simulink model "sampleModel6041_pp_1873_1_difftest"  (R2021a)
settings: Solver=VariableStepAuto  StartTime=0.0  StopTime=10.0  RelTol=1e-3
undefined symbols (not defined in the file or in its folder): Newton, Raphson
libraries: simulink x15, pid_lib x3
settings Model: Creator=O1  LastModifiedBy=user

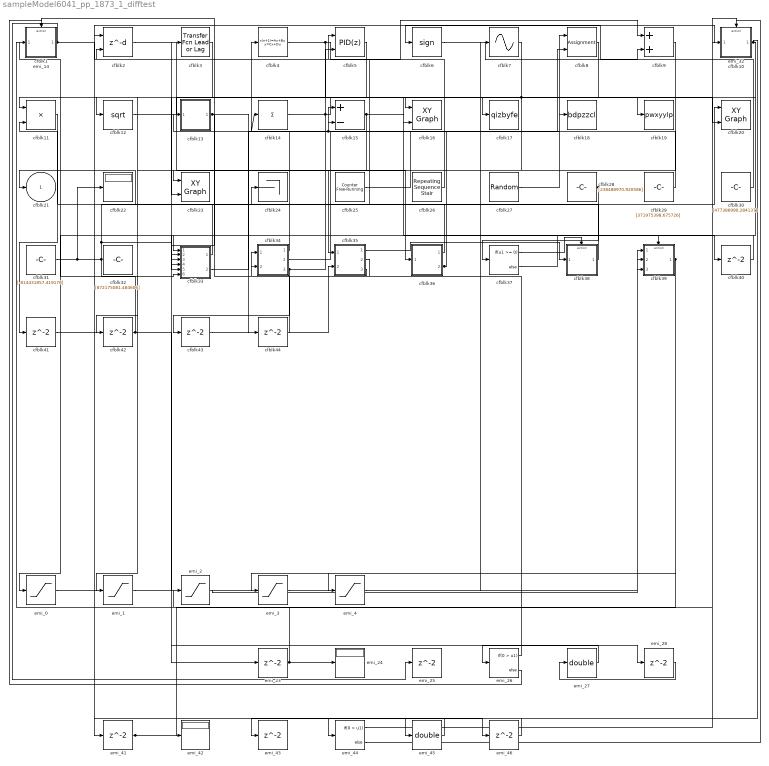
== system sampleModel6041_pp_1873_1_difftest ==
  cfblk1 : Subsystem  TreatAsAtomicUnit=on
  cfblk10 : Subsystem  TreatAsAtomicUnit=on
  cfblk11 : Product
  cfblk12 : Sqrt  SaturateOnIntegerOverflow=on
  cfblk13 : Subsystem  TreatAsAtomicUnit=on
  cfblk14 : Sum  Inputs=+
  cfblk15 : Sum  Inputs=+-
  cfblk16 : simulink/Sinks/XY Graph  xmin=-1  xmax=1  ymin=-1  ymax=1  st=-1
  cfblk17 : ToWorkspace  VariableName=qizbyfe  SaveFormat=Timeseries  SampleTime=-1
  cfblk18 : ToWorkspace  VariableName=bdpzzcl  SaveFormat=Timeseries  SampleTime=-1
  cfblk19 : ToWorkspace  VariableName=pwxyylp  SaveFormat=Timeseries  SampleTime=-1
  cfblk2 : Delay  DelayLengthSource=Input port  SampleTime=1
      settings: InputPortMap=u0,p1
  cfblk20 : simulink/Sinks/XY Graph  xmin=-1  xmax=1  ymin=-1  ymax=1  st=-1
  cfblk22 : Display
  cfblk23 : simulink/Sinks/XY Graph  xmin=-1  xmax=1  ymin=-1  ymax=1  st=-1
  cfblk24 : Terminator
  cfblk25 : simulink/Sources/Counter Free-Running  NumBits=[51.000000]  tsamp=-1
  cfblk26 : simulink/Sources/Repeating Sequence Stair  OutValues=[88415445.174803, 597697851.659731]  tsamp=-1  OutMin=[]  OutMax=[]  OutDataTypeStr=double  OutputDataTypeScalingMode=double  OutDataType=fixdt(0,8)  ConRadixGroup=Best Precision: Vector-wise  OutScaling=2^-12
  cfblk27 : RandomNumber  Mean=[16875.692149]  Variance=[94231.226590]  Seed=[933993458.000000]  SampleTime=0.1
  cfblk28 : Constant  Value=[238488970.920586]  SampleTime=1
  cfblk29 : Constant  Value=[371975398.675726]  SampleTime=1
  cfblk3 : simulink/Discrete/Transfer Fcn Lead or Lag  PoleZ=0.95  ZeroZ=0.75  ICPrevOutput=0.0  ICPrevInput=0.0  DoSatur=off
      settings: SourceProductBaseCode=SL
  cfblk30 : Constant  Value=[477386990.284137]  SampleTime=1
  cfblk31 : Constant  Value=[-814431857.419178]  SampleTime=1
  cfblk32 : Constant  Value=[872175081.484606]  SampleTime=1
  cfblk33 : Subsystem
  cfblk34 : Subsystem
  cfblk35 : Subsystem
  cfblk36 : Subsystem
  cfblk37 : If  IfExpression=u1 >= 0  SampleTime=1
  cfblk38 : Subsystem  TreatAsAtomicUnit=on
  cfblk39 : Subsystem  TreatAsAtomicUnit=on
  cfblk4 : DiscreteStateSpace
  cfblk{40..44} (5 alike) : Delay  SampleTime=1
  cfblk5 : pid_lib/PID Controller (2DOF)  Controller=PID  Form=Parallel  TimeDomain=Discrete-time  UseExternalTs=off  SampleTime=1  IntegratorMethod=Forward Euler  FilterMethod=Forward Euler  ControllerParametersSource=internal  P=1  I=1  D=0  UseFilter=on  N=100  b=1  c=1  TunerSelectOption=Transfer Function Based (PID Tuner App)  InitialConditionSource=internal  InitialConditionForIntegrator=0  InitialConditionForFilter=0  DifferentiatorICPrevScaledInput=0  ExternalReset=none  TrackingMode=off  Kt=1  LimitOutput=off  SatLimitsSource=internal  UpperSaturationLimit=inf  LowerSaturationLimit=-inf  LinearizeAsGain=off  AntiWindupMode=none  Kb=1  POutMin=[]  POutMax=[]  IOutMin=[]  IOutMax=[]  DOutMin=[]  DOutMax=[]  NOutMin=[]  NOutMax=[]  bOutMin=[]  bOutMax=[]  cOutMin=[]  cOutMax=[]  SumOutMin=[]  SumOutMax=[]  SaturationOutMin=[]  SaturationOutMax=[]  PParamMin=[]  PParamMax=[]  IParamMin=[]  IParamMax=[]  DParamMin=[]  DParamMax=[]  NParamMin=[]  NParamMax=[]  bParamMin=[]  bParamMax=[]  cParamMin=[]  cParamMax=[]  KbParamMin=[]  KbParamMax=[]  KtParamMin=[]  KtParamMax=[]  KbOutMin=[]  KbOutMax=[]  KtOutMin=[]  KtOutMax=[]  IntegratorOutMin=[]  IntegratorOutMax=[]  FilterOutMin=[]  FilterOutMax=[]  SumI1OutMin=[]  SumI1OutMax=[]  SumI2OutMin=[]  SumI2OutMax=[]  SumI3OutMin=[]  SumI3OutMax=[]  SumI4OutMin=[]  SumI4OutMax=[]  SumDOutMin=[]  SumDOutMax=[]  Sum1OutMin=[]  Sum1OutMax=[]  Sum2OutMin=[]  Sum2OutMax=[]  Sum3OutMin=[]  Sum3OutMax=[]  DifferentiatorOutMin=[]  DifferentiatorOutMax=[]  FilterDiffOutCoefMin=[]  FilterDiffOutCoefMax=[]  ReciprocalOutMin=[]  ReciprocalOutMax=[]  SumDenOutMin=[]  SumDenOutMax=[]  SumNumOutMin=[]  SumNumOutMax=[]  DivideOutMin=[]  DivideOutMax=[]  UdiffTsProdOutMin=[]  UdiffTsProdOutMax=[]  NTsProdOutMin=[]  NTsProdOutMax=[]  UintegralTsProdOutMin=[]  UintegralTsProdOutMax=[]  UngainTsProdOutMin=[]  UngainTsProdOutMax=[]  IntegratorContinuousStateAttributes=''  IntegratorStateMustResolveToSignalObject=off  IntegratorRTWStateStorageClass=Auto  FilterContinuousStateAttributes=''  FilterStateMustResolveToSignalObject=off  FilterRTWStateStorageClass=Auto  ParallelPVariant=InternalParameters  IdealPVariant=Disabled  IVariant=InternalParameters  DVariant=InternalParameters  bVariant=InternalParameters  cVariant=InternalParameters  IntegratorVariant=Discrete  SatVariant=Disabled  AWVariant=Passthrough  PCopyVariant=Disabled  TRVariant=Disabled  FdbkBlocksVariant=Forward  IdealPFdbkVariant=Disabled  SatFdbkVariant=Disabled  DerivativeFilterVariant=ForwardEulerFilter  NVariant=InternalParameters  NCopyVariant=Disabled  FilterICVariant=InternalICsFilter  IntegratorICVariant=InternalICs  ExternalResetVariant=Disabled  TRSumVariant=Passthrough  SumFdbkVariant=Disabled  SumVariant=Sum_PID  TsampFilterVariant=InternalTs  TsampNgainVariant=Passthrough  TsampIntegralVariant=Passthrough  ExternalSaturationOutDataTypeStr=Inherit: Same as second input
      settings: SourceProductBaseCode=SL
  cfblk6 : Signum
  cfblk7 : Sin  TimeSource=Use external signal  SampleTime=0
  cfblk8 : Assignment  DiagnosticForDimensions=Warning  IndexOptions=Index vector (dialog)  Indices=1  OutputSizes=1
  cfblk9 : Sum
  emi_{0..4} (5 alike) : Saturate  UpperLimit=0  LowerLimit=0  ZeroCross=off
  emi_14 : Subsystem  TreatAsAtomicUnit=on
  emi_{23,25,41,43} (4 alike) : Delay
  emi_24 : Display
  emi_26 : If  IfExpression=0 > u1
  emi_27 : DataTypeConversion  OutDataTypeStr=double
  emi_28 : Delay  InitialCondition=0
  emi_32 : Subsystem  TreatAsAtomicUnit=on
  emi_42 : Display
  emi_44 : If  IfExpression=0 > u1
  emi_45 : DataTypeConversion  OutDataTypeStr=double
  emi_46 : Delay  InitialCondition=0
  cfblk21 : Outport
  wires:
  cfblk8/1 -> cfblk11/1
  cfblk27/1 -> cfblk8/1
  cfblk7/1 -> cfblk23/1, cfblk16/2
  cfblk25/1 -> cfblk18/1
  cfblk34/1(cfblk2) -> cfblk4/1
  cfblk14/1 -> cfblk19/1, cfblk16/1
  cfblk35/1(cfblk2) -> cfblk38/1(cfblk1)
  cfblk2/1 -> cfblk36/1(cfblk1)
  cfblk30/1 -> cfblk6/1
  cfblk28/1 -> cfblk37/1, emi_0/1
  cfblk35/2(cfblk11) -> cfblk34/1(cfblk1)
  cfblk35/3(cfblk12) -> cfblk34/2(cfblk11)
  cfblk3/1 -> cfblk23/2
  cfblk4/1 -> cfblk9/1, cfblk20/2
  cfblk31/1 -> cfblk20/1, cfblk33/3(cfblk11), cfblk33/6(cfblk14), cfblk22/1
  cfblk33/1(cfblk2) -> cfblk21/1
  cfblk6/1 -> cfblk9/2
  cfblk33/2(cfblk15) -> cfblk15/1
  cfblk29/1 -> cfblk14/1, cfblk15/2
  cfblk36/1(cfblk2) -> cfblk5/1
  cfblk15/1 -> cfblk35/1(cfblk1), cfblk40/1
  cfblk38/1(cfblk2) -> cfblk11/2
  cfblk12/1 -> cfblk17/1
  cfblk34/2(cfblk12) -> cfblk8/2
  cfblk26/1 -> cfblk2/2
  cfblk34/3(cfblk13) -> cfblk5/2, cfblk43/1
  cfblk36/2(cfblk12) -> cfblk24/1, cfblk13/1(emi_9)
  cfblk37/1 -> cfblk38/Action
  cfblk37/2 -> cfblk39/Action
  cfblk40/1 -> cfblk33/1(cfblk1)
  cfblk11/1 -> cfblk41/1
  cfblk41/1 -> cfblk33/2(cfblk10)
  cfblk5/1 -> cfblk42/1
  cfblk43/1 -> cfblk35/2(cfblk10)
  cfblk44/1 -> cfblk2/1
  emi_0/1 -> cfblk7/1
  emi_1/1 -> cfblk3/1
  cfblk9/1 -> emi_1/1
  emi_2/1 -> cfblk39/1(cfblk1)
  cfblk39/1(cfblk2) -> emi_2/1, emi_3/1, emi_4/1
  emi_3/1 -> cfblk39/2(cfblk7)
  emi_4/1 -> cfblk39/3(cfblk8)
  cfblk13/1(emi_10) -> cfblk44/1, cfblk33/4(cfblk12)
  cfblk42/1 -> cfblk1/1(emi_12), emi_23/1, emi_28/1
  emi_23/1 -> emi_14/1(emi_21), emi_24/1
  emi_14/1(emi_22) -> emi_25/1
  emi_26/2 -> cfblk1/Action
  emi_26/1 -> emi_14/Action
  emi_27/1 -> emi_26/1
  emi_28/1 -> emi_27/1
  cfblk1/1(emi_13) -> cfblk10/1(emi_30), emi_41/1, emi_46/1
  cfblk10/1(emi_31) -> cfblk33/5(cfblk13), cfblk12/1
  emi_41/1 -> emi_32/1(emi_39), emi_42/1
  emi_32/1(emi_40) -> emi_43/1
  emi_44/2 -> cfblk10/Action
  emi_44/1 -> emi_32/Action
  emi_45/1 -> emi_44/1
  emi_46/1 -> emi_45/1

== system sampleModel6041_pp_1873_1_difftest/cfblk1 ==
  emi_12 : Inport
  Action Port : ActionPort  ActionPortLabel=else
  cfblk1 : Subsystem  TreatAsAtomicUnit=on
  emi_13 : Outport
  wires:
  emi_12/1 -> cfblk1/1(emi_6)
  cfblk1/1(emi_7) -> emi_13/1

== system sampleModel6041_pp_1873_1_difftest/cfblk10 ==
  emi_30 : Inport
  Action Port : ActionPort  ActionPortLabel=else
  cfblk10 : Sqrt  Operator=rSqrt  AlgorithmType=Newton-Raphson  SaturateOnIntegerOverflow=on
  emi_31 : Outport
  wires:
  emi_30/1 -> cfblk10/1
  cfblk10/1 -> emi_31/1

== system sampleModel6041_pp_1873_1_difftest/cfblk13 ==
  emi_9 : Inport  Partition=on  PartitionDimension=1  PartitionWidth=1  PartitionOffset=0
  For Each : ForEach  DisableCoverage=on
  cfblk13 : Sqrt  Operator=rSqrt  AlgorithmType=Newton-Raphson  SaturateOnIntegerOverflow=on
  emi_10 : Outport  ConcatenationDimension=1
  wires:
  emi_9/1 -> cfblk13/1
  cfblk13/1 -> emi_10/1

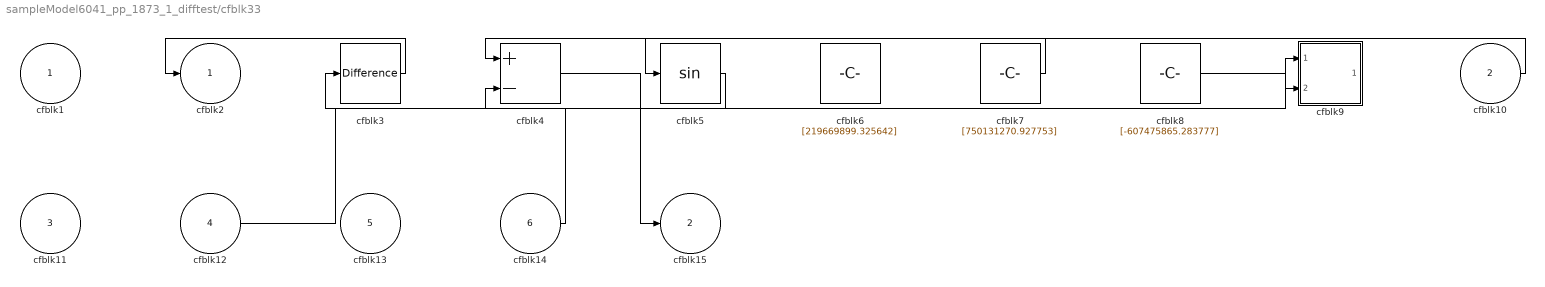
== system sampleModel6041_pp_1873_1_difftest/cfblk33 ==
  cfblk1 : Inport
  cfblk10 : Inport  Port=2
  cfblk11 : Inport  Port=3
  cfblk12 : Inport  Port=4
  cfblk13 : Inport  Port=5
  cfblk14 : Inport  Port=6
  cfblk3 : simulink/Discrete/Difference  ICPrevInput=0.0  OutMin=[]  OutMax=[]  OutDataTypeStr=Inherit: Inherit via back propagation  OutDataType=fixdt(1, 16)  OutScaling=2^-10  DoSatur=off
  cfblk4 : Sum  Inputs=+-
  cfblk5 : Trigonometry
  cfblk6 : Constant  Value=[219669899.325642]  SampleTime=1
  cfblk7 : Constant  Value=[750131270.927753]  SampleTime=1
  cfblk8 : Constant  Value=[-607475865.283777]  SampleTime=1
  cfblk9 : Subsystem
  cfblk2 : Outport
  cfblk15 : Outport  Port=2
  wires:
  cfblk12/1 -> cfblk9/1(cfblk1)
  cfblk10/1 -> cfblk5/1
  cfblk3/1 -> cfblk2/1
  cfblk7/1 -> cfblk4/1
  cfblk4/1 -> cfblk15/1
  cfblk5/1 -> cfblk4/2
  cfblk8/1 -> cfblk9/2(cfblk8)
  cfblk14/1 -> cfblk3/1

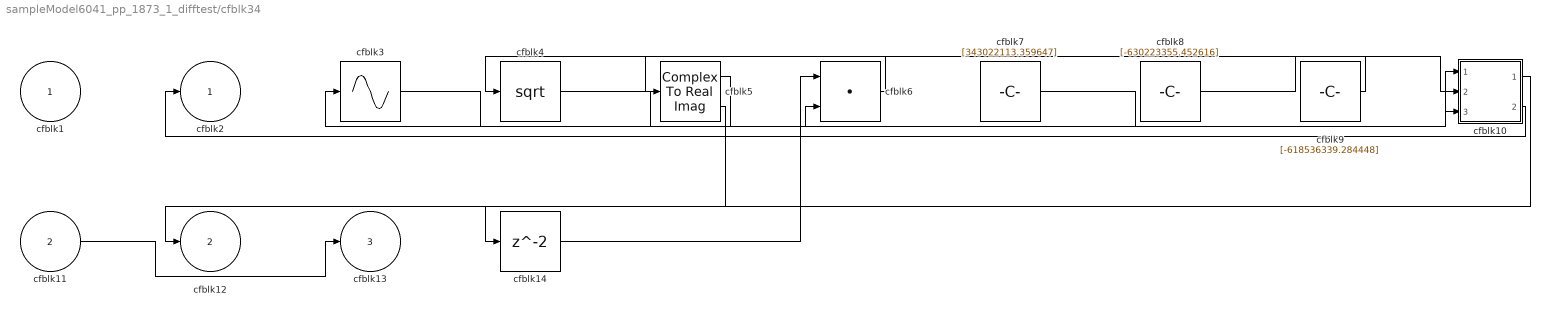
== system sampleModel6041_pp_1873_1_difftest/cfblk34 ==
  cfblk1 : Inport
  cfblk11 : Inport  Port=2
  cfblk10 : Subsystem
  cfblk14 : Delay  SampleTime=1
  cfblk3 : Sin  TimeSource=Use external signal  SampleTime=0
  cfblk4 : Sqrt  SaturateOnIntegerOverflow=on
  cfblk5 : ComplexToRealImag
  cfblk6 : DotProduct  InputSameDT=on  OutDataTypeStr=Inherit: Inherit via internal rule
  cfblk7 : Constant  Value=[343022113.359647]  SampleTime=1
  cfblk8 : Constant  Value=[-630223355.452616]  SampleTime=1
  cfblk9 : Constant  Value=[-618536339.284448]  SampleTime=1
  cfblk2 : Outport
  cfblk12 : Outport  Port=2
  cfblk13 : Outport  Port=3
  wires:
  cfblk9/1 -> cfblk4/1
  cfblk10/1(cfblk2) -> cfblk12/1
  cfblk11/1 -> cfblk13/1
  cfblk7/1 -> cfblk10/1(cfblk1)
  cfblk5/1 -> cfblk3/1
  cfblk10/2(cfblk9) -> cfblk2/1
  cfblk8/1 -> cfblk10/2(cfblk7)
  cfblk3/1 -> cfblk10/3(cfblk8)
  cfblk4/1 -> cfblk6/2
  cfblk6/1 -> cfblk5/1
  cfblk5/2 -> cfblk14/1
  cfblk14/1 -> cfblk6/1

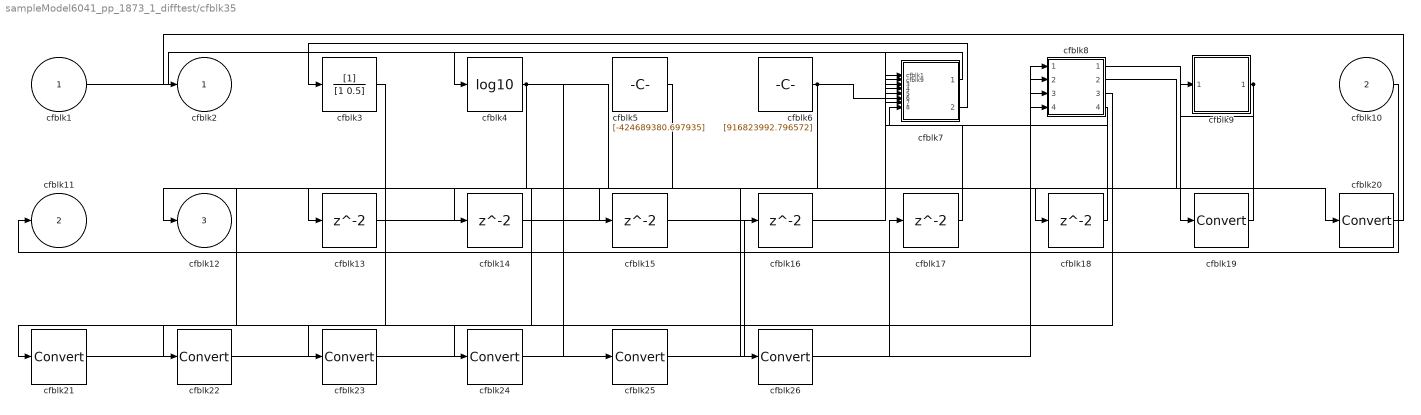
== system sampleModel6041_pp_1873_1_difftest/cfblk35 ==
  cfblk1 : Inport
  cfblk10 : Inport  Port=2
  cfblk{13..18} (6 alike) : Delay  SampleTime=1
  cfblk{19..26} (8 alike) : DataTypeConversion
  cfblk3 : DiscreteFilter  SampleTime=1
  cfblk4 : Math  Operator=log10  SaturateOnIntegerOverflow=on
  cfblk5 : Constant  Value=[-424689380.697935]  SampleTime=1
  cfblk6 : Constant  Value=[916823992.796572]  SampleTime=1
  cfblk7 : Subsystem
  cfblk8 : Subsystem
  cfblk9 : Subsystem
  cfblk2 : Outport
  cfblk11 : Outport  Port=2
  cfblk12 : Outport  Port=3
  wires:
  cfblk5/1 -> cfblk12/1
  cfblk7/1(cfblk2) -> cfblk4/1
  cfblk7/2(cfblk16) -> cfblk3/1
  cfblk4/1 -> cfblk13/1, cfblk18/1, cfblk25/1, cfblk26/1
  cfblk10/1 -> cfblk11/1
  cfblk6/1 -> cfblk7/6(cfblk13), cfblk24/1
  cfblk1/1 -> cfblk7/2(cfblk9)
  cfblk9/1(cfblk2) -> cfblk14/1, cfblk15/1
  cfblk13/1 -> cfblk7/1(cfblk1)
  cfblk14/1 -> cfblk7/3(cfblk10)
  cfblk15/1 -> cfblk7/7(cfblk14)
  cfblk16/1 -> cfblk7/4(cfblk11)
  cfblk17/1 -> cfblk7/5(cfblk12)
  cfblk18/1 -> cfblk7/8(cfblk15)
  cfblk8/1(cfblk2) -> cfblk19/1
  cfblk19/1 -> cfblk9/1(cfblk1)
  cfblk8/2(cfblk13) -> cfblk20/1
  cfblk20/1 -> cfblk2/1
  cfblk8/3(cfblk14) -> cfblk21/1
  cfblk21/1 -> cfblk16/1
  cfblk8/4(cfblk15) -> cfblk22/1
  cfblk22/1 -> cfblk17/1
  cfblk3/1 -> cfblk23/1
  cfblk23/1 -> cfblk8/1(cfblk1)
  cfblk24/1 -> cfblk8/2(cfblk10)
  cfblk25/1 -> cfblk8/3(cfblk11)
  cfblk26/1 -> cfblk8/4(cfblk12)

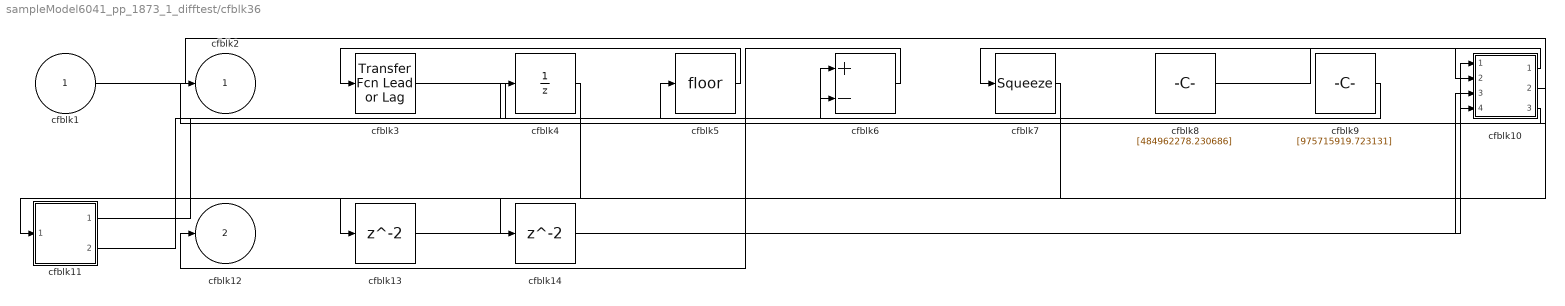
== system sampleModel6041_pp_1873_1_difftest/cfblk36 ==
  cfblk1 : Inport
  cfblk10 : Subsystem
  cfblk11 : Subsystem
  cfblk13 : Delay  SampleTime=1
  cfblk14 : Delay  SampleTime=1
  cfblk3 : simulink/Discrete/Transfer Fcn Lead or Lag  PoleZ=0.95  ZeroZ=0.75  ICPrevOutput=0.0  ICPrevInput=0.0  DoSatur=off
      settings: SourceProductBaseCode=SL
  cfblk4 : UnitDelay  HasFrameUpgradeWarning=on
  cfblk5 : Rounding
  cfblk6 : Sum  Inputs=+-
  cfblk7 : Squeeze
  cfblk8 : Constant  Value=[484962278.230686]  SampleTime=1
  cfblk9 : Constant  Value=[975715919.723131]  SampleTime=1
  cfblk2 : Outport
  cfblk12 : Outport  Port=2
  wires:
  cfblk10/1(cfblk2) -> cfblk7/1
  cfblk9/1 -> cfblk6/1
  cfblk11/1(cfblk2) -> cfblk5/1
  cfblk5/1 -> cfblk3/1
  cfblk6/1 -> cfblk12/1
  cfblk1/1 -> cfblk10/1(cfblk1)
  cfblk10/2(cfblk13) -> cfblk11/1(cfblk1)
  cfblk8/1 -> cfblk10/2(cfblk10)
  cfblk3/1 -> cfblk6/2
  cfblk11/2(cfblk8) -> cfblk4/1
  cfblk10/3(cfblk14) -> cfblk2/1
  cfblk7/1 -> cfblk13/1
  cfblk13/1 -> cfblk10/4(cfblk12)
  cfblk4/1 -> cfblk14/1
  cfblk14/1 -> cfblk10/3(cfblk11)

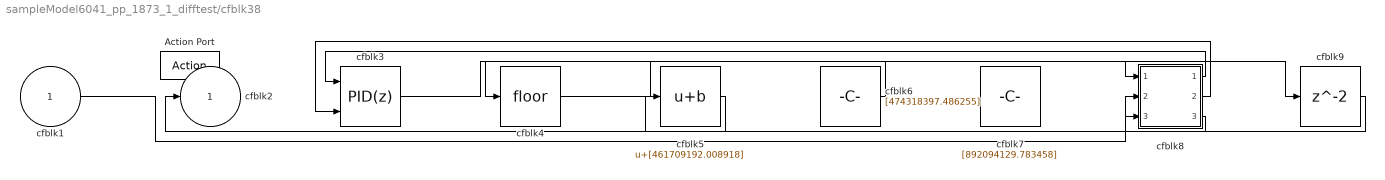
== system sampleModel6041_pp_1873_1_difftest/cfblk38 ==
  cfblk1 : Inport
  Action Port : ActionPort  ActionPortLabel=if(u1 >= 0)
  cfblk3 : pid_lib/PID Controller (2DOF)  Controller=PID  Form=Parallel  TimeDomain=Discrete-time  UseExternalTs=off  SampleTime=-1  IntegratorMethod=Forward Euler  FilterMethod=Forward Euler  ControllerParametersSource=internal  P=1  I=1  D=0  UseFilter=on  N=100  b=1  c=1  TunerSelectOption=Transfer Function Based (PID Tuner App)  InitialConditionSource=internal  InitialConditionForIntegrator=0  InitialConditionForFilter=0  DifferentiatorICPrevScaledInput=0  ExternalReset=none  TrackingMode=off  Kt=1  LimitOutput=off  SatLimitsSource=internal  UpperSaturationLimit=inf  LowerSaturationLimit=-inf  LinearizeAsGain=off  AntiWindupMode=none  Kb=1  POutMin=[]  POutMax=[]  IOutMin=[]  IOutMax=[]  DOutMin=[]  DOutMax=[]  NOutMin=[]  NOutMax=[]  bOutMin=[]  bOutMax=[]  cOutMin=[]  cOutMax=[]  SumOutMin=[]  SumOutMax=[]  SaturationOutMin=[]  SaturationOutMax=[]  PParamMin=[]  PParamMax=[]  IParamMin=[]  IParamMax=[]  DParamMin=[]  DParamMax=[]  NParamMin=[]  NParamMax=[]  bParamMin=[]  bParamMax=[]  cParamMin=[]  cParamMax=[]  KbParamMin=[]  KbParamMax=[]  KtParamMin=[]  KtParamMax=[]  KbOutMin=[]  KbOutMax=[]  KtOutMin=[]  KtOutMax=[]  IntegratorOutMin=[]  IntegratorOutMax=[]  FilterOutMin=[]  FilterOutMax=[]  SumI1OutMin=[]  SumI1OutMax=[]  SumI2OutMin=[]  SumI2OutMax=[]  SumI3OutMin=[]  SumI3OutMax=[]  SumI4OutMin=[]  SumI4OutMax=[]  SumDOutMin=[]  SumDOutMax=[]  Sum1OutMin=[]  Sum1OutMax=[]  Sum2OutMin=[]  Sum2OutMax=[]  Sum3OutMin=[]  Sum3OutMax=[]  DifferentiatorOutMin=[]  DifferentiatorOutMax=[]  FilterDiffOutCoefMin=[]  FilterDiffOutCoefMax=[]  ReciprocalOutMin=[]  ReciprocalOutMax=[]  SumDenOutMin=[]  SumDenOutMax=[]  SumNumOutMin=[]  SumNumOutMax=[]  DivideOutMin=[]  DivideOutMax=[]  UdiffTsProdOutMin=[]  UdiffTsProdOutMax=[]  NTsProdOutMin=[]  NTsProdOutMax=[]  UintegralTsProdOutMin=[]  UintegralTsProdOutMax=[]  UngainTsProdOutMin=[]  UngainTsProdOutMax=[]  IntegratorContinuousStateAttributes=''  IntegratorStateMustResolveToSignalObject=off  IntegratorRTWStateStorageClass=Auto  FilterContinuousStateAttributes=''  FilterStateMustResolveToSignalObject=off  FilterRTWStateStorageClass=Auto  ParallelPVariant=InternalParameters  IdealPVariant=Disabled  IVariant=InternalParameters  DVariant=InternalParameters  bVariant=InternalParameters  cVariant=InternalParameters  IntegratorVariant=Discrete  SatVariant=Disabled  AWVariant=Passthrough  PCopyVariant=Disabled  TRVariant=Disabled  FdbkBlocksVariant=Forward  IdealPFdbkVariant=Disabled  SatFdbkVariant=Disabled  DerivativeFilterVariant=ForwardEulerFilter  NVariant=InternalParameters  NCopyVariant=Disabled  FilterICVariant=InternalICsFilter  IntegratorICVariant=InternalICs  ExternalResetVariant=Disabled  TRSumVariant=Passthrough  SumFdbkVariant=Disabled  SumVariant=Sum_PID  TsampFilterVariant=InternalTs  TsampNgainVariant=Passthrough  TsampIntegralVariant=Passthrough  ExternalSaturationOutDataTypeStr=Inherit: Same as second input
      settings: SourceProductBaseCode=SL
  cfblk4 : Rounding
  cfblk5 : Bias  Bias=[461709192.008918]
  cfblk6 : Constant  Value=[474318397.486255]  SampleTime=1
  cfblk7 : Constant  Value=[892094129.783458]  SampleTime=1
  cfblk8 : Subsystem
  cfblk9 : Delay
  cfblk2 : Outport
  wires:
  cfblk6/1 -> cfblk4/1
  cfblk5/1 -> cfblk2/1
  cfblk8/1(cfblk2) -> cfblk3/1
  cfblk4/1 -> cfblk8/1(cfblk1)
  cfblk1/1 -> cfblk8/2(cfblk9)
  cfblk8/2(cfblk11) -> cfblk3/2
  cfblk8/3(cfblk12) -> cfblk5/1
  cfblk3/1 -> cfblk9/1
  cfblk9/1 -> cfblk8/3(cfblk10)

== system sampleModel6041_pp_1873_1_difftest/cfblk39 ==
  cfblk1 : Inport
  cfblk7 : Inport  Port=2
  cfblk8 : Inport  Port=3
  Action Port : ActionPort  ActionPortLabel=else
  cfblk3 : Rounding
  cfblk5 : Constant  Value=[330239103.049017]  SampleTime=1
  cfblk6 : Constant  Value=[710880281.477537]  SampleTime=1
  cfblk2 : Outport
  wires:
  cfblk7/1 -> cfblk3/1
  cfblk5/1 -> cfblk2/1

== system sampleModel6041_pp_1873_1_difftest/emi_14 ==
  emi_21 : Inport
  Action Port : ActionPort  ActionPortLabel=if(0 > u1)
  emi_18 : MinMax
  emi_19 : MinMax
  emi_20 : MinMax
  emi_22 : Outport
  wires:
  emi_21/1 -> emi_18/1
  emi_18/1 -> emi_19/1
  emi_19/1 -> emi_20/1

== system sampleModel6041_pp_1873_1_difftest/emi_32 ==
  emi_39 : Inport
  Action Port : ActionPort  ActionPortLabel=if(0 > u1)
  emi_36 : Gain
  emi_37 : Math  SaturateOnIntegerOverflow=on
  emi_38 : Trigonometry
  emi_40 : Outport
  wires:
  emi_39/1 -> emi_36/1
  emi_36/1 -> emi_37/1
  emi_37/1 -> emi_38/1

== system sampleModel6041_pp_1873_1_difftest/cfblk1/cfblk1 ==
  emi_6 : Inport  Partition=on  PartitionDimension=1  PartitionWidth=1  PartitionOffset=0
  For Each : ForEach  DisableCoverage=on
  cfblk1 : simulink/Discrete/Tapped Delay  vinit=0.0  samptime=-1  NumDelays=1  DelayOrder=Oldest  includeCurrent=off
  emi_7 : Outport  ConcatenationDimension=1
  wires:
  cfblk1/1 -> emi_7/1
  emi_6/1 -> cfblk1/1

== system sampleModel6041_pp_1873_1_difftest/cfblk33/cfblk9 ==
  cfblk1 : Inport
  cfblk8 : Inport  Port=2
  cfblk3 : Product  Inputs=*
  cfblk4 : Product  Inputs=*
  cfblk5 : Gain  Gain=[-8146701.246174]
  cfblk6 : Sum  Inputs=--
  cfblk7 : Constant  Value=[-996140999.230012]  SampleTime=1
  cfblk2 : Outport
  wires:
  cfblk8/1 -> cfblk5/1
  cfblk1/1 -> cfblk3/1
  cfblk5/1 -> cfblk6/1
  cfblk3/1 -> cfblk6/2
  cfblk7/1 -> cfblk4/1
  cfblk6/1 -> cfblk2/1

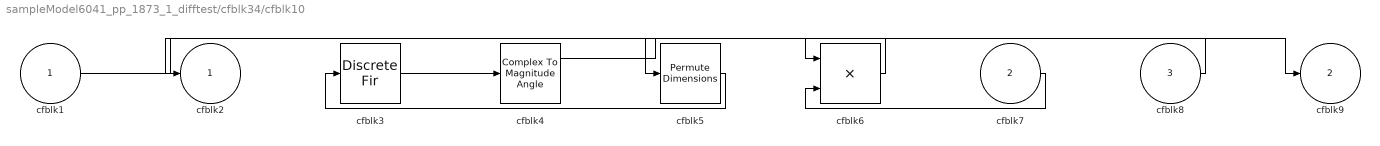
== system sampleModel6041_pp_1873_1_difftest/cfblk34/cfblk10 ==
  cfblk1 : Inport
  cfblk7 : Inport  Port=2
  cfblk8 : Inport  Port=3
  cfblk3 : DiscreteFir  SampleTime=1
  cfblk4 : ComplexToMagnitudeAngle
  cfblk5 : PermuteDimensions
  cfblk6 : Product  Inputs=**
  cfblk2 : Outport
  cfblk9 : Outport  Port=2
  wires:
  cfblk3/1 -> cfblk4/1
  cfblk8/1 -> cfblk6/1
  cfblk1/1 -> cfblk5/1
  cfblk5/1 -> cfblk3/1
  cfblk7/1 -> cfblk6/2
  cfblk6/1 -> cfblk2/1
  cfblk4/1 -> cfblk9/1

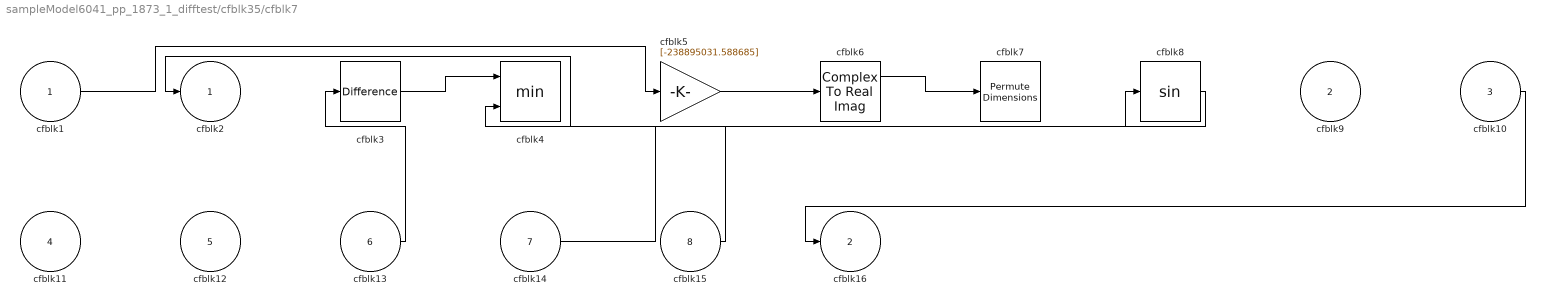
== system sampleModel6041_pp_1873_1_difftest/cfblk35/cfblk7 ==
  cfblk1 : Inport
  cfblk9 : Inport  Port=2
  cfblk10 : Inport  Port=3
  cfblk11 : Inport  Port=4
  cfblk12 : Inport  Port=5
  cfblk13 : Inport  Port=6
  cfblk14 : Inport  Port=7
  cfblk15 : Inport  Port=8
  cfblk3 : simulink/Discrete/Difference  ICPrevInput=0.0  OutMin=[]  OutMax=[]  OutDataTypeStr=Inherit: Inherit via back propagation  OutDataType=fixdt(1, 16)  OutScaling=2^-10  DoSatur=off
  cfblk4 : MinMax  Inputs=2
  cfblk5 : Gain  Gain=[-238895031.588685]
  cfblk6 : ComplexToRealImag
  cfblk7 : PermuteDimensions
  cfblk8 : Trigonometry
  cfblk2 : Outport
  cfblk16 : Outport  Port=2
  wires:
  cfblk3/1 -> cfblk4/1
  cfblk10/1 -> cfblk16/1
  cfblk13/1 -> cfblk3/1
  cfblk15/1 -> cfblk2/1
  cfblk1/1 -> cfblk5/1
  cfblk5/1 -> cfblk6/1
  cfblk8/1 -> cfblk4/2
  cfblk6/1 -> cfblk7/1
  cfblk14/1 -> cfblk8/1

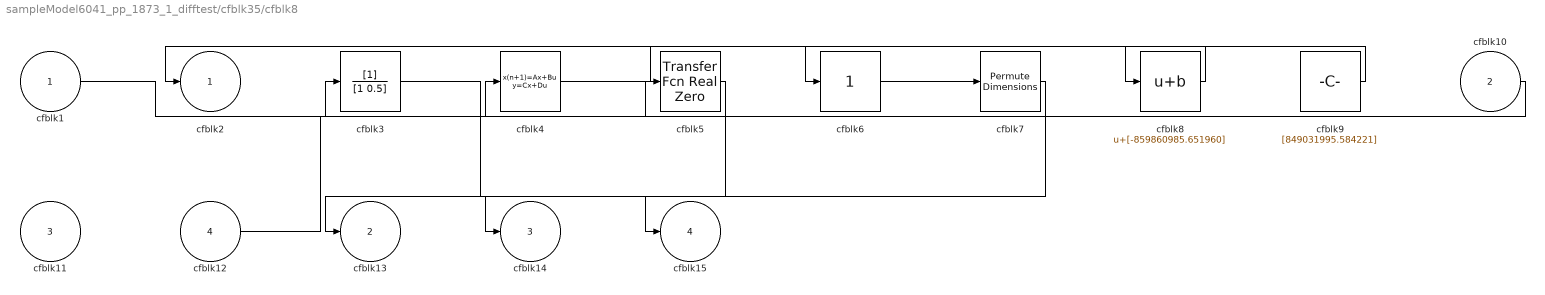
== system sampleModel6041_pp_1873_1_difftest/cfblk35/cfblk8 ==
  cfblk1 : Inport
  cfblk10 : Inport  Port=2
  cfblk11 : Inport  Port=3
  cfblk12 : Inport  Port=4
  cfblk3 : DiscreteFilter  SampleTime=1
  cfblk4 : DiscreteStateSpace
  cfblk5 : simulink/Discrete/Transfer Fcn Real Zero  ZeroZ=0.75  ICPrevInput=0.0  DoSatur=off
      settings: SourceProductBaseCode=SL
  cfblk6 : simulink/Math Operations/Slider Gain  gain=1  low=0  high=2
  cfblk7 : PermuteDimensions
  cfblk8 : Bias  Bias=[-859860985.651960]
  cfblk9 : Constant  Value=[849031995.584221]  SampleTime=1
  cfblk2 : Outport
  cfblk13 : Outport  Port=2
  cfblk14 : Outport  Port=3
  cfblk15 : Outport  Port=4
  wires:
  cfblk9/1 -> cfblk2/1
  cfblk10/1 -> cfblk4/1
  cfblk5/1 -> cfblk13/1
  cfblk3/1 -> cfblk15/1
  cfblk4/1 -> cfblk8/1
  cfblk8/1 -> cfblk6/1
  cfblk7/1 -> cfblk14/1
  cfblk1/1 -> cfblk3/1
  cfblk6/1 -> cfblk7/1
  cfblk12/1 -> cfblk5/1

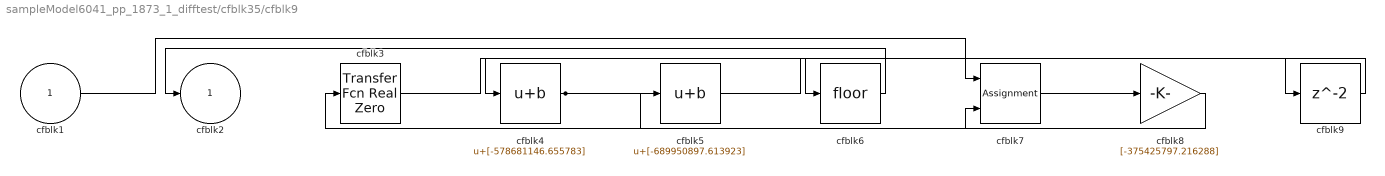
== system sampleModel6041_pp_1873_1_difftest/cfblk35/cfblk9 ==
  cfblk1 : Inport
  cfblk3 : simulink/Discrete/Transfer Fcn Real Zero  ZeroZ=0.75  ICPrevInput=0.0  DoSatur=off
      settings: SourceProductBaseCode=SL
  cfblk4 : Bias  Bias=[-578681146.655783]
  cfblk5 : Bias  Bias=[-689950897.613923]
  cfblk6 : Rounding
  cfblk7 : Assignment  DiagnosticForDimensions=Warning  IndexOptions=Index vector (dialog)  Indices=1  OutputSizes=1
  cfblk8 : Gain  Gain=[-375425797.216288]
  cfblk9 : Delay  SampleTime=1
  cfblk2 : Outport
  wires:
  cfblk4/1 -> cfblk5/1, cfblk7/2
  cfblk8/1 -> cfblk3/1
  cfblk6/1 -> cfblk2/1
  cfblk1/1 -> cfblk7/1
  cfblk3/1 -> cfblk6/1
  cfblk7/1 -> cfblk8/1
  cfblk5/1 -> cfblk9/1
  cfblk9/1 -> cfblk4/1

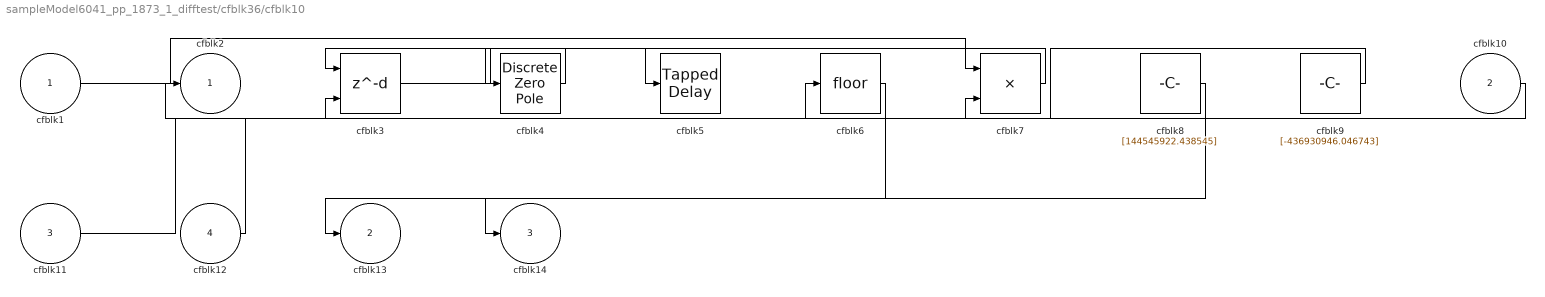
== system sampleModel6041_pp_1873_1_difftest/cfblk36/cfblk10 ==
  cfblk1 : Inport
  cfblk10 : Inport  Port=2
  cfblk11 : Inport  Port=3
  cfblk12 : Inport  Port=4
  cfblk3 : Delay  DelayLengthSource=Input port  SampleTime=1
      settings: InputPortMap=u0,p1
  cfblk4 : DiscreteZeroPole  Poles=[0 0.5]  Gain=1
  cfblk5 : simulink/Discrete/Tapped Delay  vinit=0.0  samptime=-1  NumDelays=1  DelayOrder=Oldest  includeCurrent=off
  cfblk6 : Rounding
  cfblk7 : Product  Inputs=**
  cfblk8 : Constant  Value=[144545922.438545]  SampleTime=1
  cfblk9 : Constant  Value=[-436930946.046743]  SampleTime=1
  cfblk2 : Outport
  cfblk13 : Outport  Port=2
  cfblk14 : Outport  Port=3
  wires:
  cfblk3/1 -> cfblk5/1
  cfblk8/1 -> cfblk13/1
  cfblk11/1 -> cfblk6/1
  cfblk1/1 -> cfblk7/1
  cfblk6/1 -> cfblk14/1
  cfblk9/1 -> cfblk7/2
  cfblk4/1 -> cfblk3/1
  cfblk7/1 -> cfblk4/1
  cfblk10/1 -> cfblk3/2
  cfblk12/1 -> cfblk2/1

== system sampleModel6041_pp_1873_1_difftest/cfblk36/cfblk11 ==
  cfblk1 : Inport
  cfblk3 : DiscreteTransferFcn  SampleTime=1
  cfblk4 : Delay  SampleTime=1
  cfblk5 : pid_lib/PID Controller  Controller=PID  Form=Parallel  TimeDomain=Discrete-time  UseExternalTs=off  SampleTime=1  IntegratorMethod=Forward Euler  FilterMethod=Forward Euler  ControllerParametersSource=internal  P=1  I=1  D=0  UseFilter=on  N=100  TunerSelectOption=Transfer Function Based (PID Tuner App)  InitialConditionSource=internal  InitialConditionForIntegrator=0  InitialConditionForFilter=0  DifferentiatorICPrevScaledInput=0  ExternalReset=none  TrackingMode=off  Kt=1  LimitOutput=off  SatLimitsSource=internal  UpperSaturationLimit=inf  LowerSaturationLimit=-inf  LinearizeAsGain=off  AntiWindupMode=none  Kb=1  POutMin=[]  POutMax=[]  IOutMin=[]  IOutMax=[]  DOutMin=[]  DOutMax=[]  NOutMin=[]  NOutMax=[]  SumOutMin=[]  SumOutMax=[]  SaturationOutMin=[]  SaturationOutMax=[]  PParamMin=[]  PParamMax=[]  IParamMin=[]  IParamMax=[]  DParamMin=[]  DParamMax=[]  NParamMin=[]  NParamMax=[]  KbParamMin=[]  KbParamMax=[]  KtParamMin=[]  KtParamMax=[]  KbOutMin=[]  KbOutMax=[]  KtOutMin=[]  KtOutMax=[]  IntegratorOutMin=[]  IntegratorOutMax=[]  FilterOutMin=[]  FilterOutMax=[]  SumI1OutMin=[]  SumI1OutMax=[]  SumI2OutMin=[]  SumI2OutMax=[]  SumI3OutMin=[]  SumI3OutMax=[]  SumI4OutMin=[]  SumI4OutMax=[]  SumDOutMin=[]  SumDOutMax=[]  DifferentiatorOutMin=[]  DifferentiatorOutMax=[]  FilterDiffOutCoefMin=[]  FilterDiffOutCoefMax=[]  ReciprocalOutMin=[]  ReciprocalOutMax=[]  SumDenOutMin=[]  SumDenOutMax=[]  SumNumOutMin=[]  SumNumOutMax=[]  DivideOutMin=[]  DivideOutMax=[]  UdiffTsProdOutMin=[]  UdiffTsProdOutMax=[]  NTsProdOutMin=[]  NTsProdOutMax=[]  UintegralTsProdOutMin=[]  UintegralTsProdOutMax=[]  UngainTsProdOutMin=[]  UngainTsProdOutMax=[]  IntegratorContinuousStateAttributes=''  IntegratorStateMustResolveToSignalObject=off  IntegratorRTWStateStorageClass=Auto  FilterContinuousStateAttributes=''  FilterStateMustResolveToSignalObject=off  FilterRTWStateStorageClass=Auto  ParallelPVariant=InternalParameters  IdealPVariant=Disabled  IVariant=InternalParameters  DVariant=InternalParameters  IntegratorVariant=Discrete  SatVariant=Disabled  AWVariant=Passthrough  PCopyVariant=Disabled  TRVariant=Disabled  FdbkBlocksVariant=Forward  IdealPFdbkVariant=Disabled  SatFdbkVariant=Disabled  DerivativeFilterVariant=ForwardEulerFilter  NVariant=InternalParameters  NCopyVariant=Disabled  FilterICVariant=InternalICsFilter  IntegratorICVariant=InternalICs  ExternalResetVariant=Disabled  TRSumVariant=Passthrough  SumFdbkVariant=Disabled  SumVariant=Sum_PID  TsampFilterVariant=InternalTs  TsampNgainVariant=Passthrough  TsampIntegralVariant=Passthrough  ExternalSaturationOutDataTypeStr=Inherit: Same as second input
  cfblk6 : Squeeze
  cfblk7 : Sqrt  SaturateOnIntegerOverflow=on
  cfblk9 : Delay  SampleTime=1
  cfblk2 : Outport
  cfblk8 : Outport  Port=2
  wires:
  cfblk3/1 -> cfblk7/1
  cfblk4/1 -> cfblk6/1
  cfblk6/1 -> cfblk5/1, cfblk2/1
  cfblk1/1 -> cfblk4/1
  cfblk5/1 -> cfblk8/1
  cfblk7/1 -> cfblk9/1
  cfblk9/1 -> cfblk3/1

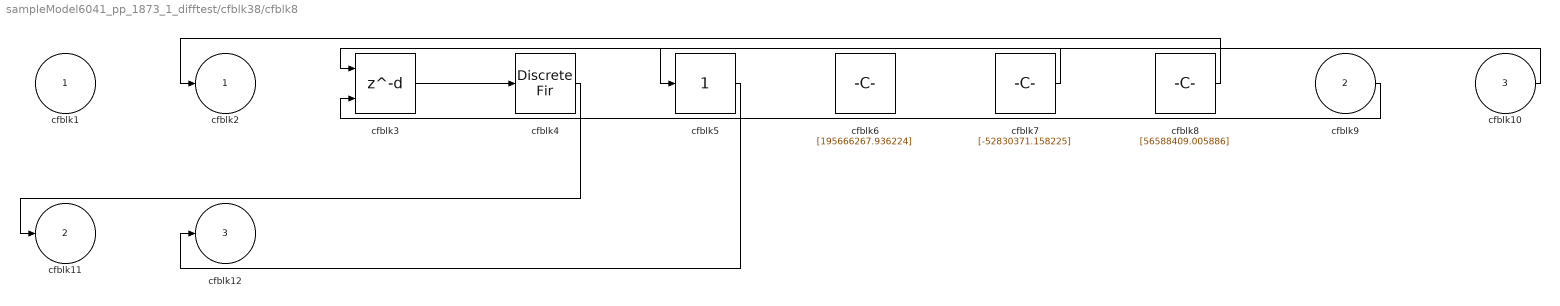
== system sampleModel6041_pp_1873_1_difftest/cfblk38/cfblk8 ==
  cfblk1 : Inport
  cfblk9 : Inport  Port=2
  cfblk10 : Inport  Port=3
  cfblk3 : Delay  DelayLengthSource=Input port
      settings: InputPortMap=u0,p1
  cfblk4 : DiscreteFir
  cfblk5 : simulink/Math Operations/Slider Gain  gain=1  low=0  high=2
  cfblk6 : Constant  Value=[195666267.936224]  SampleTime=1
  cfblk7 : Constant  Value=[-52830371.158225]  SampleTime=1
  cfblk8 : Constant  Value=[56588409.005886]  SampleTime=1
  cfblk2 : Outport
  cfblk11 : Outport  Port=2
  cfblk12 : Outport  Port=3
  wires:
  cfblk4/1 -> cfblk11/1
  cfblk7/1 -> cfblk5/1
  cfblk8/1 -> cfblk2/1
  cfblk5/1 -> cfblk12/1
  cfblk3/1 -> cfblk4/1
  cfblk10/1 -> cfblk3/1
  cfblk9/1 -> cfblk3/2
